simulink model "tubemodel2"  (Simulink 7.3)
settings: Solver=ode45  StartTime=0.0  StopTime=100.0  RelTol=1e-3
libraries: simulink x2, dspsrcs4 x1
settings Model: Creator=Hörnstein  LastModifiedBy=Hörnstein

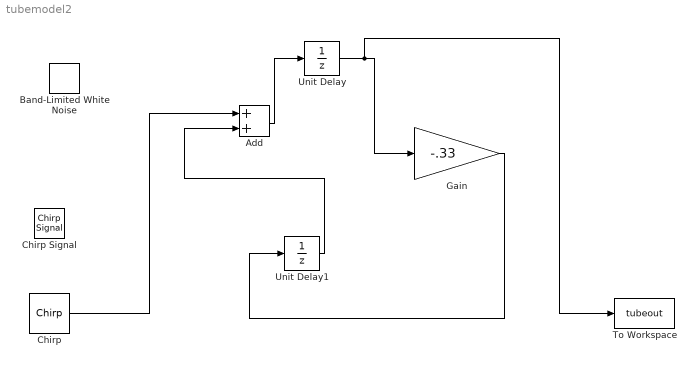
== system tubemodel2 ==
  Add : Sum  OutDataType=fixdt(1, 16)  OutScaling=2^-10
  Band-Limited White Noise : simulink/Sources/Band-Limited White Noise  SystemSampleTime=-1  Cov=[0.1]  Ts=0.1  seed=[23341]
  Chirp : dspsrcs4/Chirp  sweep=Linear  mode=Unidirectional  f0=0  f1=4000  t1=1  Tsweep=1  phase=0  Ts=1/2000  spf=1  datatype=Double
  Chirp Signal : simulink/Sources/Chirp Signal  SystemSampleTime=-1  f1=0  T=20  f2=2000
  Gain : Gain  Gain=-.33  ParameterDataType=fixdt(1, 16)  ParameterScaling=2^0  OutDataType=fixdt(1, 16)  OutScaling=2^0
  To Workspace : ToWorkspace  VariableName=tubeout  SampleTime=-1  SaveFormat=Array
  Unit Delay : UnitDelay  SampleTime=-1
  Unit Delay1 : UnitDelay  SampleTime=-1
  wires:
  Gain/1 -> Unit Delay1/1
  Unit Delay1/1 -> Add/2
  Add/1 -> Unit Delay/1
  Unit Delay/1 -> Gain/1, To Workspace/1
  Chirp/1 -> Add/1
